simulink model "lab2ex4"  (R2023b)
settings: Solver=VariableStepAuto  StartTime=-3  StopTime=5  RelTol=1e-3
libraries: SignalEditorBlockLib x2
settings Model: Creator=shaanyadav  LastModifiedBy=shaanyadav

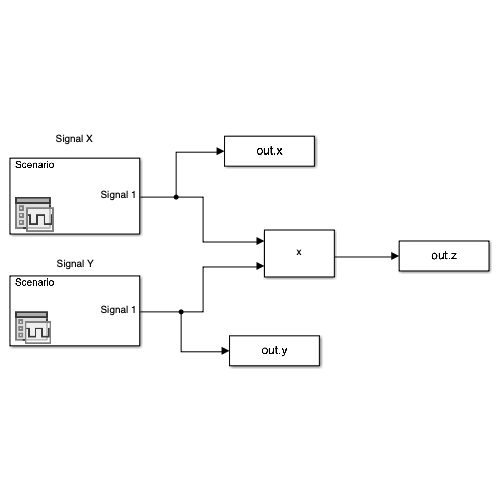
[thumbnail: Simulink's stored preview of the top-level diagram]
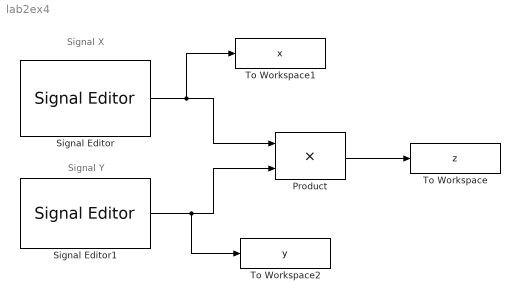
== system lab2ex4 ==
  note: Signal X
  note: Signal Y
  Product : Product
  Signal Editor : SignalEditorBlockLib/Signal Editor  FileName=signal1.mat  ActiveScenario=Scenario  ActiveSignal=Signal 1  IsBus=off  OutputBusObjectStr=Bus: BusObject  SampleTime=0  OutputAfterFinalValue=Setting to zero  Unit=inherit  PreserveSignalName=on  ApplySigPropsToAllScenarios=on  ApplySigPropsToAllSignals=off
  Signal Editor1 : SignalEditorBlockLib/Signal Editor  FileName=signal2.mat  ActiveScenario=Scenario  ActiveSignal=Signal 1  IsBus=off  OutputBusObjectStr=Bus: BusObject  SampleTime=0  OutputAfterFinalValue=Setting to zero  Unit=inherit  PreserveSignalName=on  ApplySigPropsToAllScenarios=on  ApplySigPropsToAllSignals=off
  To Workspace : ToWorkspace  VariableName=z  SampleTime=-1
  To Workspace1 : ToWorkspace  VariableName=x  SampleTime=-1
  To Workspace2 : ToWorkspace  VariableName=y  SampleTime=-1
  wires:
  Signal Editor/1 -> To Workspace1/1, Product/1
  Signal Editor1/1 -> To Workspace2/1, Product/2
  Product/1 -> To Workspace/1
